simulink model "SAD_PROJECT"  (R2023b)
settings: Solver=ode5  StartTime=0.0  StopTime=5920  FixedStep=0.01  RelTol=1e-10  AbsTol=1e-11
values from neighbouring files (symbols this model uses):
  A = [0,  (1-K_yaw)*n, 0, -K_yaw*n^2,  0,   0 ... (first row only)    [SAD_CALLER.m]
  A_0 = A_B_LVLH*A_LVLH_ECI_0    [SAD_CALLER.m]    (also in veriAxilsym.m = eye(3))
  A_slew_B_LVLH = rot_matrix(deg2rad(-15.3),1)*rot_matrix(deg2rad(0),2)*rot_matrix(deg2rad(0),3)*eye(3)    [SAD_CALLER.m]
  alpha_mount_hs = 0.15    [SAD_CALLER.m]
  alpha_mount_ss = -0.5    [SAD_CALLER.m]
  B = [1/I(1,1),0,0 ... (first row only)    [SAD_CALLER.m]
  C = [0,0,0,1,0,0 ... (first row only)    [SAD_CALLER.m]
  correct_g = [5.7   7.4   0      0     0 ... (first row only)    [SAD_CALLER.m]    (also in veriAxilsym.m)
  correct_h = [  0  -25.9     0       0      0 ... (first row only)    [SAD_CALLER.m]    (also in veriAxilsym.m)
  d_cm_rw = 0.00000005    (= 5e-08)    [SAD_CALLER.m]
  d_cmsc_rw = 0.003    [SAD_CALLER.m]
  f = @(F) -F+e*sinh(F)+F_s-e*sinh(F_s)-M_h    [SAD_CALLER.m]
  FOV = 34    [SAD_CALLER.m]
  g_nm = [-29404.8 -1450.9     0      0     0 ... (first row only)    [SAD_CALLER.m]    (also in veriAxilsym.m)
  h_nm = [  0  4652.5      0      0       0 ... (first row only)    [SAD_CALLER.m]    (also in veriAxilsym.m)
  I = I_a+diag([0,4*M_a*x_cm^2,4*M_a*x_cm^2])+I_c+diag([0,M_c*d_cc_cm^2,M_c*d_cc_cm^2])+I_p+diag([0,6*M_p*(d_cc+d_cc_cm)^2,6*M_p*(d_cc-d_cc_cm)^2])    [SAD_CALLER.m]    (also in veriAxilsym.m = diag(I))
  I_r = 9.55e-5    (= 9.55e-05)    [SAD_CALLER.m]
  Inv_I = inv(I)    [SAD_CALLER.m]    (also in veriAxilsym.m = pinv(I))
  inv_R = inv(R)    [SAD_CALLER.m]
  J2 = 1.082626925638815e-3    (= 0.00108262692564)    [SAD_CALLER.m]    (also in veriAxilsym.m)
  K = [ -0.4323    0.0000   -0.0000   -0.0105    0.0000   -0.0000 ... (first row only)    [SAD_CALLER.m]
  L = [  0.0663    0.0001    0.0068 ... (first row only)    [SAD_CALLER.m]
  M_brake = 0.0002    [SAD_CALLER.m]
  M_rw = 0.2    [SAD_CALLER.m]    (also in veriAxilsym.m)
  m_sc_body = [1;1;1]*10e-3*M_tot/sqrt(3)    [SAD_CALLER.m]    (also in veriAxilsym.m)
  maneuver = input('type of maneuver, 1 for nadir pointing, 2 for de-tumbling, 3 for slew ')    [SAD_CALLER.m]
  mu_E = 3.986004418e5    (= 398600.4418)    [SAD_CALLER.m]    (also in veriAxilsym.m = 398600)
  mu_S = 1.327124400e11    (= 132712440000)    [SAD_CALLER.m]
  n = 2*pi/T    [SAD_CALLER.m]
  om_rw_0 = [0,0,0]    [SAD_CALLER.m]
  omega_E = 2*pi/(24*60*60)    (= 7.27220521664e-05)    [SAD_CALLER.m]    (also in veriAxilsym.m)
  omega_sc_0 = [0,0,n]    [SAD_CALLER.m]    (also in veriAxilsym.m = [0; 0; 0])
  pinv_R_xy = pinv(R_xy)    [SAD_CALLER.m]
  pinv_R_xz = pinv(R_xz)    [SAD_CALLER.m]
  pinv_R_yz = pinv(R_yz)    [SAD_CALLER.m]
  R = [cos(angle),-sin(angle),0;sin(angle),cos(angle),0;0,0,1]    [SAD_CALLER.m]    (also in veriAxilsym.m = 6378.1363)
  R_E_eqtr = 6378.1363    [SAD_CALLER.m]    (also in veriAxilsym.m)
  R_x = R(:,1)    [SAD_CALLER.m]
  R_y = R(:,2)    [SAD_CALLER.m]
  R_z = R(:,3)    [SAD_CALLER.m]
  rr_Esc_0 = s(end,(1:3))'    [SAD_CALLER.m]    (also in veriAxilsym.m = [7070.6; 0; 0])
  RR_x = [R_x,R_rad_x_1',R_rad_x_2']    [SAD_CALLER.m]
  RR_y = [R_y,R_rad_y_1',R_rad_y_2']    [SAD_CALLER.m]
  RR_z = [R_z,R_rad_z_1',R_rad_z_2']    [SAD_CALLER.m]
  smith_norm = zeros(4,5)    [SAD_CALLER.m]    (also in veriAxilsym.m)
  theta_G0 = mod(theta_G_Winter_solstice+omega_E*t_elapsed,2*pi)    [SAD_CALLER.m]    (also in veriAxilsym.m)
  vv_Esc_0 = s(end,(4:6))'    [SAD_CALLER.m]    (also in veriAxilsym.m = [0; 7.4338; 0])
undefined symbols (not defined in the file or in its folder): omega_0, rr_ES_0, vv_ES_0
libraries: matrix_library x24, simulink_extras x9, simulink x5
(part 1 of 2)
settings Model: Creator=WinUser  LastModifiedBy=a1pab

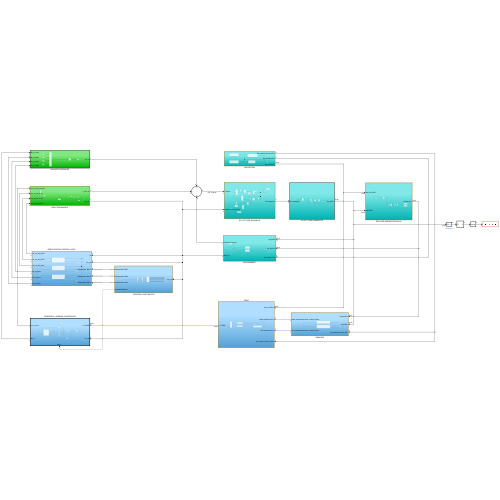
[thumbnail: Simulink's stored preview of the top-level diagram]
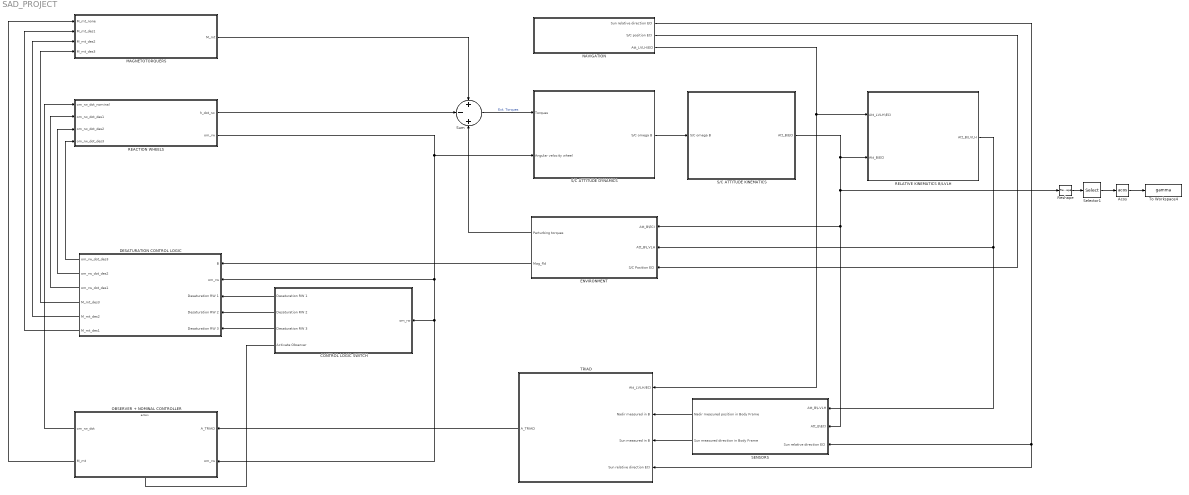
== system SAD_PROJECT ==
  Acos : Trigonometry  Operator=acos
  CONTROL LOGIC SWITCH : Subsystem
  DESATURATION CONTROL LOGIC : Subsystem
  ENVIRONMENT : Subsystem
  MAGNETOTORQUERS : Subsystem
  NAVIGATION : Subsystem
  OBSERVER + NOMINAL CONTROLLER : Subsystem  TreatAsAtomicUnit=on
  REACTION WHEELS : Subsystem
  RELATIVE KINEMATICS B/LVLH : Subsystem
  Reshape : Reshape
  S/C ATTITUDE DYNAMICS : Subsystem
  S/C ATTITUDE KINEMATICS : Subsystem
  SENSORS : Subsystem
  Selector1 : Selector  InputPortWidth=9  IndexOptions=Index vector (dialog)  Indices=[1,5,9]  OutputSizes=1
  Sum : Sum  Inputs=+-+
  TRIAD : Subsystem
  To Workspace4 : ToWorkspace  VariableName=gamma  SampleTime=-1
      settings: Save2DSignal=2-D array (concatenate along first dimension)
  wires:
  Sum/1 -> S/C ATTITUDE DYNAMICS/1(Torques)  "Ext. Torques"
  S/C ATTITUDE KINEMATICS/1(Att_B\ECI) -> Reshape/1, SENSORS/2(Att_B\ECI), ENVIRONMENT/1(Att_B\ECI), RELATIVE KINEMATICS B/LVLH/2(Att_B\ECI)
  ENVIRONMENT/1(Perturbing torques) -> Sum/3
  RELATIVE KINEMATICS B/LVLH/1(Att_B\LVLH) -> ENVIRONMENT/2(Att_B\LVLH), SENSORS/1(Att_B\LVLH)
  NAVIGATION/1(Sun relative direction ECI) -> TRIAD/4(Sun relative direction ECI), SENSORS/3(Sun relative direction ECI)
  NAVIGATION/3(Att_LVLH\ECI) -> TRIAD/1(Att_LVLH/ECI), RELATIVE KINEMATICS B/LVLH/1(Att_LVLH\ECI)
  NAVIGATION/2(S/C position ECI) -> ENVIRONMENT/3(S/C Position ECI)
  REACTION WHEELS/1(h_dot_rw) -> Sum/2
  ENVIRONMENT/2(Mag_fld) -> DESATURATION CONTROL LOGIC/1(B)
  SENSORS/1(Nadir measured position in Body Frame) -> TRIAD/2(Nadir measured in B)
  SENSORS/2(Sun measured direction in Body Frame) -> TRIAD/3(Sun measured in B)
  REACTION WHEELS/2(om_rw) -> OBSERVER + NOMINAL CONTROLLER/2(om_rw), CONTROL LOGIC SWITCH/1(om_rw), DESATURATION CONTROL LOGIC/2(om_rw), S/C ATTITUDE DYNAMICS/2(Angular velocity wheel)
  CONTROL LOGIC SWITCH/4(Activate Observer) -> OBSERVER + NOMINAL CONTROLLER/Action
  CONTROL LOGIC SWITCH/1(Desaturation RW 1) -> DESATURATION CONTROL LOGIC/3(Desaturation RW 1)
  CONTROL LOGIC SWITCH/2(Desaturation RW 2) -> DESATURATION CONTROL LOGIC/4(Desaturation RW 2)
  CONTROL LOGIC SWITCH/3(Desaturation RW 3) -> DESATURATION CONTROL LOGIC/5(Desaturation RW 3)
  OBSERVER + NOMINAL CONTROLLER/1(om_rw_dot) -> REACTION WHEELS/1(om_rw_dot_nominal)
  DESATURATION CONTROL LOGIC/3(om_rw_dot_des1) -> REACTION WHEELS/2(om_rw_dot_des1)
  DESATURATION CONTROL LOGIC/2(om_rw_dot_des2) -> REACTION WHEELS/3(om_rw_dot_des2)
  DESATURATION CONTROL LOGIC/1(om_rw_dot_des3) -> REACTION WHEELS/4(om_rw_dot_des3)
  DESATURATION CONTROL LOGIC/4(M_mt_des3) -> MAGNETOTORQUERS/4(M_mt_des3)
  DESATURATION CONTROL LOGIC/5(M_mt_des2) -> MAGNETOTORQUERS/3(M_mt_des2)
  DESATURATION CONTROL LOGIC/6(M_mt_des1) -> MAGNETOTORQUERS/2(M_mt_des1)
  MAGNETOTORQUERS/1(M_mt) -> Sum/1
  OBSERVER + NOMINAL CONTROLLER/2(M_mt) -> MAGNETOTORQUERS/1(M_mt_none)
  TRIAD/1(A_TRIAD) -> OBSERVER + NOMINAL CONTROLLER/1(A_TRIAD)
  S/C ATTITUDE DYNAMICS/1(S/C omega B) -> S/C ATTITUDE KINEMATICS/1(S/C omega B)
  Selector1/1 -> Acos/1
  Reshape/1 -> Selector1/1
  Acos/1 -> To Workspace4/1

== system SAD_PROJECT/CONTROL LOGIC SWITCH ==
  om_rw : Inport
  Abs : Abs  SaturateOnIntegerOverflow=off
  Abs1 : Abs  SaturateOnIntegerOverflow=off
  Abs2 : Abs  SaturateOnIntegerOverflow=off
  Demux : Demux  Outputs=3
  If : If  NumInputs=3  IfExpression=u1 == 1  ElseIfExpressions=u2== 1,u3==1
  Relay : Relay  OnSwitchValue=500  OffSwitchValue=100
  Relay1 : Relay  OnSwitchValue=500  OffSwitchValue=100
  Relay2 : Relay  OnSwitchValue=500  OffSwitchValue=100
  Desaturation RW 1 : Outport
  Desaturation RW 2 : Outport  Port=2
  Desaturation RW 3 : Outport  Port=3
  Activate Observer : Outport  Port=4
  wires:
  Demux/3 -> Abs2/1
  Demux/1 -> Abs/1
  Abs/1 -> Relay/1
  Demux/2 -> Abs1/1
  Abs2/1 -> Relay2/1
  Relay1/1 -> If/2
  Abs1/1 -> Relay1/1
  Relay/1 -> If/1
  Relay2/1 -> If/3
  If/1 -> Desaturation RW 1/1
  If/4 -> Activate Observer/1
  If/2 -> Desaturation RW 2/1
  om_rw/1 -> Demux/1
  If/3 -> Desaturation RW 3/1

== system SAD_PROJECT/DESATURATION CONTROL LOGIC ==
  B : Inport
  om_rw : Inport  Port=2
  Desaturation RW 1 : Inport  Port=3
  Desaturation RW 2 : Inport  Port=4
  Desaturation RW 3 : Inport  Port=5
  RW 1 Desaturation : Subsystem
  RW 2 Desaturation : Subsystem
  RW 3 Desaturation : Subsystem
  om_rw_dot_des3 : Outport
  om_rw_dot_des2 : Outport  Port=2
  om_rw_dot_des1 : Outport  Port=3
  M_mt_des3 : Outport  Port=4
  M_mt_des2 : Outport  Port=5
  M_mt_des1 : Outport  Port=6
  wires:
  Desaturation RW 1/1 -> RW 1 Desaturation/Action
  B/1 -> RW 3 Desaturation/1(B), RW 2 Desaturation/1(B), RW 1 Desaturation/1(B)
  Desaturation RW 2/1 -> RW 2 Desaturation/Action
  Desaturation RW 3/1 -> RW 3 Desaturation/Action
  om_rw/1 -> RW 3 Desaturation/2(om_rw), RW 2 Desaturation/2(om_rw), RW 1 Desaturation/2(om_rw)
  RW 1 Desaturation/1(M_mt) -> M_mt_des1/1
  RW 1 Desaturation/2(om_rw_dot) -> om_rw_dot_des1/1
  RW 2 Desaturation/1(M_mt) -> M_mt_des2/1
  RW 2 Desaturation/2(om_rw_dot) -> om_rw_dot_des2/1
  RW 3 Desaturation/1(M_mt) -> M_mt_des3/1
  RW 3 Desaturation/2(om_rw_dot) -> om_rw_dot_des3/1

== system SAD_PROJECT/ENVIRONMENT ==
  Att_B\ECI : Inport
  Att_B\LVLH : Inport  Port=2
  S/C Position ECI : Inport  Port=3
  Gravity Gradient : Subsystem
  Magnetic Torque : Subsystem
  Sum : Sum  Inputs=+|+
  To Workspace1 : ToWorkspace  VariableName=ext_perturbations  SampleTime=-1
  Perturbing torques : Outport
  Mag_fld : Outport  Port=2
  wires:
  S/C Position ECI/1 -> Gravity Gradient/2(S/C Position), Magnetic Torque/1("[km]")
  Att_B\ECI/1 -> Magnetic Torque/2(True Attitude B\N)
  Att_B\LVLH/1 -> Gravity Gradient/1(Att_B\L)
  Gravity Gradient/1(GG_Torque) -> Sum/1
  Sum/1 -> To Workspace1/1, Perturbing torques/1
  Magnetic Torque/1(MF_Torque) -> Sum/2
  Magnetic Torque/2(Mag_fld) -> Mag_fld/1

== system SAD_PROJECT/MAGNETOTORQUERS ==
  M_mt_none : Inport
  M_mt_des1 : Inport  Port=2
  M_mt_des2 : Inport  Port=3
  M_mt_des3 : Inport  Port=4
  Merge1 : Merge  Inputs=4
  Rate Limiter : RateLimiter  RisingSlewLimit=0.001  FallingSlewLimit=-0.001
  M_mt : Outport
  wires:
  Rate Limiter/1 -> M_mt/1
  Merge1/1 -> Rate Limiter/1
  M_mt_none/1 -> Merge1/1
  M_mt_des3/1 -> Merge1/4
  M_mt_des2/1 -> Merge1/3
  M_mt_des1/1 -> Merge1/2

== system SAD_PROJECT/NAVIGATION ==
  LVLH Kinematics : Subsystem
  S/C Orbit propagation : Subsystem
  Subsystem : Subsystem
  Sun orbit propagation : Subsystem
  Sun relative direction ECI : Outport
  S/C position ECI : Outport  Port=2
  Att_LVLH\ECI : Outport  Port=3
  wires:
  S/C Orbit propagation/1(S/C Posiion ECI) -> Subsystem/2(S/C position in ECI), S/C position ECI/1, LVLH Kinematics/1(position)
  Subsystem/1(Sun relative direction in ECI) -> Sun relative direction ECI/1
  Sun orbit propagation/1(Sun position in ECI) -> Subsystem/1(Sun position in ECI)
  S/C Orbit propagation/2(S/C Velocity ECI) -> LVLH Kinematics/2(velocity)  "[km/s]"
  LVLH Kinematics/1(Att_LVLH\ECI) -> Att_LVLH\ECI/1

== system SAD_PROJECT/OBSERVER + NOMINAL CONTROLLER ==
  A_TRIAD : Inport
  om_rw : Inport  Port=2
  Action Port : ActionPort  ActionPortLabel=else
  Gain : Gain  Gain=A  Multiplication=Matrix(K*u) (u vector)
  Gain1 : Gain  Gain=B  Multiplication=Matrix(K*u) (u vector)
  Gain2 : Gain  Gain=C  Multiplication=Matrix(K*u) (u vector)
  Gain3 : Gain  Gain=L  Multiplication=Matrix(K*u) (u vector)
  Integrator : Integrator
  NOMINAL CONTROL : Subsystem
  Reshape1 : Reshape
  Selector1 : Selector  InputPortWidth=9  IndexOptions=Index vector (dialog)  Indices=[8,3,4]  OutputSizes=1
  Sum2 : Sum  Inputs=|+-
  Sum4 : Sum  Inputs=+++
  om_rw_dot : Outport
  M_mt : Outport  Port=2
  wires:
  Sum4/1 -> Integrator/1
  NOMINAL CONTROL/1(u) -> Gain1/1
  Gain1/1 -> Sum4/1
  Gain3/1 -> Sum4/2
  Gain/1 -> Sum4/3
  Sum2/1 -> Gain3/1
  Gain2/1 -> Sum2/2
  Integrator/1 -> Gain/1, Gain2/1, NOMINAL CONTROL/1(x_hat)  "x_hat"
  om_rw/1 -> NOMINAL CONTROL/2(om_rw)
  NOMINAL CONTROL/2(om_rw_dot) -> om_rw_dot/1
  NOMINAL CONTROL/3(M_mt) -> M_mt/1
  A_TRIAD/1 -> Reshape1/1
  Reshape1/1 -> Selector1/1
  Selector1/1 -> Sum2/1  "[alpha_x,alpha_y,alpha_z"

== system SAD_PROJECT/REACTION WHEELS ==
  om_rw_dot_nominal : Inport
  om_rw_dot_des1 : Inport  Port=2
  om_rw_dot_des2 : Inport  Port=3
  om_rw_dot_des3 : Inport  Port=4
  Band-Limited White Noise : simulink/Sources/Band-Limited White Noise  Cov=[0.1]  Ts=0.1  seed=[23341]
  Constant1 : Constant  Value=om_rw_0
  Constant5 : Constant  Value=[I_r;I_r;I_r]
  Constant7 : Constant  Value=R
  Gain : Gain  Gain=1.74
  Integrator : Integrator  InitialConditionSource=external
  Matrix Multiply4 : Product
  Matrix Multiply7 : Product  Multiplication=Matrix(*)
  Merge : Merge  Inputs=4
  Rate Limiter1 : RateLimiter  RisingSlewLimit=0.001  FallingSlewLimit=-0.001  SampleTimeMode=inherited
  Saturation : Saturate  UpperLimit=125  LowerLimit=-125
  Subsystem1 : Subsystem
  Sum : Sum  Inputs=++|
  Sum1 : Sum  Inputs=|+-
  To Workspace : ToWorkspace  VariableName=rw_perturbations  SaveFormat=Timeseries  SampleTime=-1
  Transfer Fcn : TransferFcn  Denominator=[10 1]
  h_dot_rw : Outport
  om_rw : Outport  Port=2
  wires:
  Constant5/1 -> Matrix Multiply4/1
  Constant7/1 -> Matrix Multiply7/1
  Sum/1 -> Subsystem1/1(om_rw), om_rw/1  "om_rw"
  Merge/1 -> Saturation/1  "om_dot_rw"
  Matrix Multiply4/1 -> Matrix Multiply7/2  "h_dot_rw"
  Constant1/1 -> Integrator/2
  Matrix Multiply7/1 -> Rate Limiter1/1
  om_rw_dot_nominal/1 -> Merge/1  "om_dot_rw"
  Rate Limiter1/1 -> Sum1/1
  Saturation/1 -> Matrix Multiply4/2, Integrator/1
  Band-Limited White Noise/1 -> Gain/1
  Gain/1 -> Transfer Fcn/1
  Integrator/1 -> Sum/2  "om_rw"
  Subsystem1/1(disturbance torque) -> To Workspace/1, Sum1/2
  Sum1/1 -> h_dot_rw/1
  Transfer Fcn/1 -> Sum/1
  om_rw_dot_des1/1 -> Merge/2
  om_rw_dot_des2/1 -> Merge/3
  om_rw_dot_des3/1 -> Merge/4

== system SAD_PROJECT/RELATIVE KINEMATICS B//LVLH ==
  Att_LVLH\ECI : Inport
  Att_B\ECI : Inport  Port=2
  Acos : Trigonometry  Operator=acos
  Demux : Demux  Outputs=2
  Matrix Multiply1 : Product  Multiplication=Matrix(*)
  Radians to Degrees : simulink_extras/Transformations/Radians to Degrees
  Reshape : Reshape
  Selector : Selector  InputPortWidth=9  IndexOptions=Index vector (dialog)  Indices=[1,9]  OutputSizes=1
  To Workspace2 : ToWorkspace  VariableName=alpha_x  SampleTime=-1
      settings: Save2DSignal=2-D array (concatenate along first dimension)
  To Workspace3 : ToWorkspace  VariableName=alpha_z  SampleTime=-1
      settings: Save2DSignal=2-D array (concatenate along first dimension)
  Transpose1 : Math  Operator=transpose
  Att_B\LVLH : Outport
  wires:
  Transpose1/1 -> Matrix Multiply1/2  "A_N\\L"
  Matrix Multiply1/1 -> Reshape/1, Att_B\LVLH/1  "A B\\L"
  Att_B\ECI/1 -> Matrix Multiply1/1
  Att_LVLH\ECI/1 -> Transpose1/1
  Demux/2 -> To Workspace3/1
  Demux/1 -> To Workspace2/1
  Selector/1 -> Acos/1
  Reshape/1 -> Selector/1
  Radians to Degrees/1 -> Demux/1
  Acos/1 -> Radians to Degrees/1

== system SAD_PROJECT/S//C ATTITUDE DYNAMICS ==
  note: omega
  Torques : Inport
  Angular velocity wheel : Inport  Port=2
  Constant : Constant  Value=omega_sc_0
  Constant1 : Constant  Value=I  VectorParams1D=off
  Constant2 : Constant  Value=R
  Constant3 : Constant  Value=Inv_I  VectorParams1D=off
  Constant4 : Constant  Value=[I_r;I_r;I_r]
  Cross Product : matrix_library/Cross Product
  Integrator : Integrator  InitialConditionSource=external  InitialCondition=omega_0
  Matrix Multiply : Product  Multiplication=Matrix(*)
  Matrix Multiply1 : Product
  Matrix Multiply2 : Product  Multiplication=Matrix(*)
  Product : Product  Multiplication=Matrix(*)
  Sum : Sum  Inputs=|+-
  Sum1 : Sum  Inputs=|++
  To Workspace : ToWorkspace  VariableName=omega_rw  SampleTime=-1
  To Workspace4 : ToWorkspace  VariableName=omega_sc  SampleTime=-1
  S/C omega B : Outport
  wires:
  Constant3/1 -> Matrix Multiply/1
  Constant/1 -> Integrator/2
  Sum/1 -> Matrix Multiply/2
  Cross Product/1 -> Sum/2
  Integrator/1 -> To Workspace4/1, S/C omega B/1, Cross Product/1, Product/2
  Constant1/1 -> Product/1
  Matrix Multiply/1 -> Integrator/1
  Torques/1 -> Sum/1
  Angular velocity wheel/1 -> To Workspace/1, Matrix Multiply1/2
  Constant2/1 -> Matrix Multiply2/1
  Product/1 -> Sum1/1
  Sum1/1 -> Cross Product/2
  Matrix Multiply2/1 -> Sum1/2
  Constant4/1 -> Matrix Multiply1/1
  Matrix Multiply1/1 -> Matrix Multiply2/2

== system SAD_PROJECT/S//C ATTITUDE KINEMATICS ==
  S/C omega B : Inport
  1st order orthon. : Subsystem
  Angular velocity tensor : Subsystem
  Constant3 : Constant  Value=A_0
  Gain : Gain  Gain=-1
  Integrator1 : Integrator  InitialConditionSource=external  InitialCondition=omega_0
  Matrix Multiply : Product  Multiplication=Matrix(*)
  Att_B\ECI : Outport
  wires:
  Constant3/1 -> Integrator1/2
  S/C omega B/1 -> Angular velocity tensor/1(In1)  "omega B\\N"
  1st order orthon./1(Out1) -> Att_B\ECI/1, Matrix Multiply/2  "True Attitude B\\N"
  Integrator1/1 -> 1st order orthon./1(In1)
  Matrix Multiply/1 -> Integrator1/1
  Gain/1 -> Matrix Multiply/1
  Angular velocity tensor/1(Out1) -> Gain/1

== system SAD_PROJECT/SENSORS ==
  Att_B\LVLH : Inport
  Att_B\ECI : Inport  Port=2
  Sun relative direction ECI : Inport  Port=3
  Horizon Sensor : Subsystem
  Sun Sensor : Subsystem
  Nadir measured position in Body Frame : Outport
  Sun measured direction in Body Frame : Outport  Port=2
  wires:
  Att_B\ECI/1 -> Sun Sensor/1(Attitude B\ECI)
  Att_B\LVLH/1 -> Horizon Sensor/1(Attitude B\L)
  Sun relative direction ECI/1 -> Sun Sensor/2(Sun relative direction in ECI)
  Horizon Sensor/1(Nadir measured position in Body Frame) -> Nadir measured position in Body Frame/1
  Sun Sensor/1(Sun measured direction in Body Frame) -> Sun measured direction in Body Frame/1

== system SAD_PROJECT/TRIAD ==
  Att_LVLH/ECI : Inport
  Nadir measured in B : Inport  Port=2
  Sun measured in B : Inport  Port=3
  Sun relative direction ECI : Inport  Port=4
  Constant : Constant  Value=[1;0;0]
  Matrix Multiply : Product  Multiplication=Matrix(*)
  Subsystem : Subsystem
  Subsystem1 : Subsystem
  Subsystem2 : Subsystem
  Zero-Order Hold : ZeroOrderHold  SampleTime=0.2
  A_TRIAD : Outport
  wires:
  Sun relative direction ECI/1 -> Subsystem1/2(Sun relative direction ECI)
  Matrix Multiply/1 -> A_TRIAD/1
  Att_LVLH/ECI/1 -> Subsystem1/1(Att_LVLH/ECI)
  Nadir measured in B/1 -> Subsystem/1(a)
  Sun measured in B/1 -> Subsystem/2(b)
  Subsystem/1(Measures in Body) -> Matrix Multiply/1
  Constant/1 -> Subsystem2/1(Nadir in LVLH)  "Nadir in LVLH"
  Subsystem1/1(Sun direction in LVLH) -> Subsystem2/2(Sun in LVLH)  "Sun in LVLH"
  Subsystem2/1(Out1) -> Zero-Order Hold/1
  Zero-Order Hold/1 -> Matrix Multiply/2

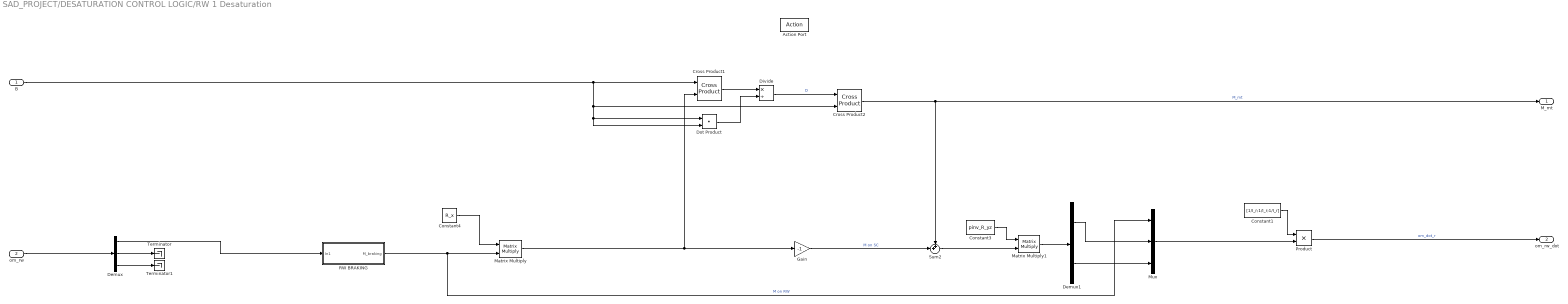
== system SAD_PROJECT/DESATURATION CONTROL LOGIC/RW 1 Desaturation ==
  B : Inport
  om_rw : Inport  Port=2
  Action Port : ActionPort  ActionPortLabel=if(u1 == 1)
  Constant1 : Constant  Value=[1/I_r;1/I_r;1/I_r]
  Constant3 : Constant  Value=pinv_R_yz
  Constant4 : Constant  Value=R_x
  Cross Product1 : matrix_library/Cross Product
  Cross Product2 : matrix_library/Cross Product
  Demux : Demux  Outputs=3
  Demux1 : Demux  Outputs=2
  Divide : Product  Inputs=*/
  Dot Product : DotProduct  OutDataTypeStr=Inherit: Inherit via internal rule
  Gain : Gain  Gain=-1
  Matrix Multiply : Product  Multiplication=Matrix(*)
  Matrix Multiply1 : Product  Multiplication=Matrix(*)
  Mux : Mux  Inputs=3
  Product : Product
  RW BRAKING : Subsystem
  Sum2 : Sum  Inputs=++|
  Terminator : Terminator
  Terminator1 : Terminator
  M_mt : Outport
  om_rw_dot : Outport  Port=2
  wires:
  Product/1 -> om_rw_dot/1  "om_dot_r"
  Cross Product2/1 -> Sum2/1, M_mt/1  "M_mt"
  Demux/3 -> Terminator1/1
  Constant3/1 -> Matrix Multiply1/1
  Matrix Multiply1/1 -> Demux1/1
  Constant4/1 -> Matrix Multiply/1
  Mux/1 -> Product/2
  Dot Product/1 -> Divide/2
  Demux1/2 -> Mux/3
  Demux/1 -> RW BRAKING/1(In1)
  Sum2/1 -> Matrix Multiply1/2
  Constant1/1 -> Product/1
  Divide/1 -> Cross Product2/1  "D"
  B/1 -> Dot Product/1, Dot Product/2, Cross Product2/2, Cross Product1/1
  RW BRAKING/1(M_braking) -> Mux/1, Matrix Multiply/2  "M on RW"
  om_rw/1 -> Demux/1
  Matrix Multiply/1 -> Gain/1, Cross Product1/2
  Cross Product1/1 -> Divide/1
  Gain/1 -> Sum2/2  "M on SC"
  Demux/2 -> Terminator/1
  Demux1/1 -> Mux/2

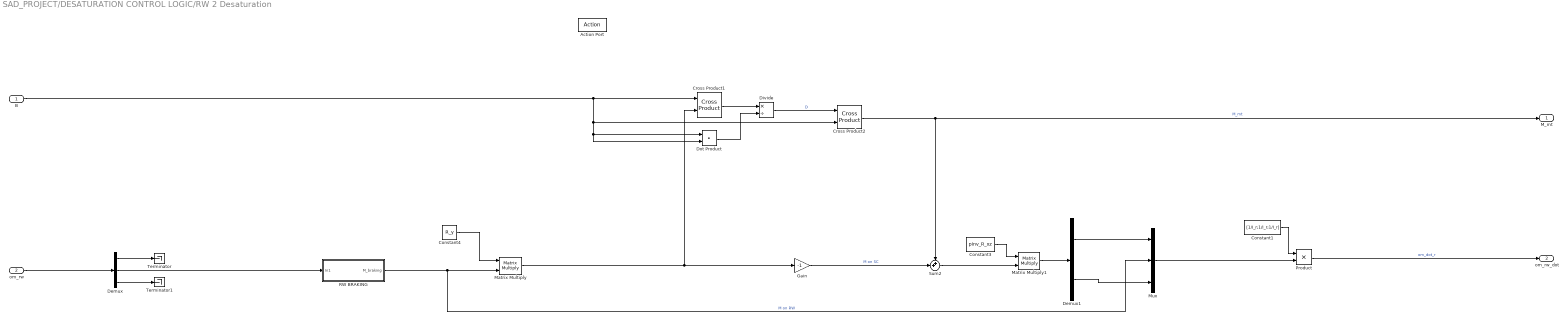
== system SAD_PROJECT/DESATURATION CONTROL LOGIC/RW 2 Desaturation ==
  B : Inport
  om_rw : Inport  Port=2
  Action Port : ActionPort  ActionPortLabel=elseif(u2== 1)
  Constant1 : Constant  Value=[1/I_r;1/I_r;1/I_r]
  Constant3 : Constant  Value=pinv_R_xz
  Constant4 : Constant  Value=R_y
  Cross Product1 : matrix_library/Cross Product
  Cross Product2 : matrix_library/Cross Product
  Demux : Demux  Outputs=3
  Demux1 : Demux  Outputs=2
  Divide : Product  Inputs=*/
  Dot Product : DotProduct  OutDataTypeStr=Inherit: Inherit via internal rule
  Gain : Gain  Gain=-1
  Matrix Multiply : Product  Multiplication=Matrix(*)
  Matrix Multiply1 : Product  Multiplication=Matrix(*)
  Mux : Mux  Inputs=3
  Product : Product
  RW BRAKING : Subsystem
  Sum2 : Sum  Inputs=++|
  Terminator : Terminator
  Terminator1 : Terminator
  M_mt : Outport
  om_rw_dot : Outport  Port=2
  wires:
  Demux1/1 -> Mux/1
  Cross Product2/1 -> Sum2/1, M_mt/1  "M_mt"
  B/1 -> Dot Product/1, Dot Product/2, Cross Product2/2, Cross Product1/1
  Dot Product/1 -> Divide/2
  Constant4/1 -> Matrix Multiply/1
  Divide/1 -> Cross Product2/1  "D"
  Cross Product1/1 -> Divide/1
  RW BRAKING/1(M_braking) -> Mux/2, Matrix Multiply/2  "M on RW"
  Demux1/2 -> Mux/3
  Gain/1 -> Sum2/2  "M on SC"
  Sum2/1 -> Matrix Multiply1/2
  Constant3/1 -> Matrix Multiply1/1
  om_rw/1 -> Demux/1
  Demux/2 -> RW BRAKING/1(In1)
  Demux/3 -> Terminator1/1
  Demux/1 -> Terminator/1
  Constant1/1 -> Product/1
  Product/1 -> om_rw_dot/1  "om_dot_r"
  Mux/1 -> Product/2
  Matrix Multiply1/1 -> Demux1/1
  Matrix Multiply/1 -> Gain/1, Cross Product1/2

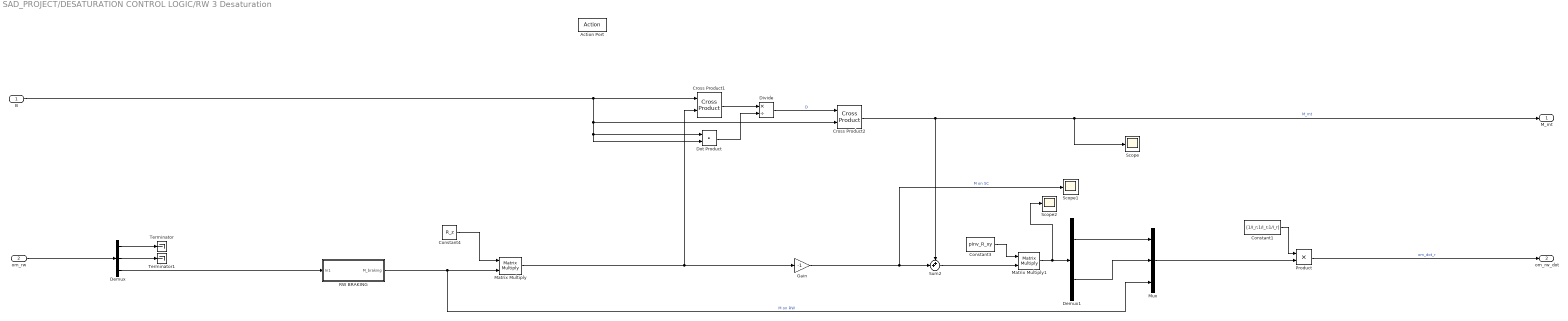
== system SAD_PROJECT/DESATURATION CONTROL LOGIC/RW 3 Desaturation ==
  B : Inport
  om_rw : Inport  Port=2
  Action Port : ActionPort  ActionPortLabel=elseif(u3==1)
  Constant1 : Constant  Value=[1/I_r;1/I_r;1/I_r]
  Constant3 : Constant  Value=pinv_R_xy
  Constant4 : Constant  Value=R_z
  Cross Product1 : matrix_library/Cross Product
  Cross Product2 : matrix_library/Cross Product
  Demux : Demux  Outputs=3
  Demux1 : Demux  Outputs=2
  Divide : Product  Inputs=*/
  Dot Product : DotProduct  OutDataTypeStr=Inherit: Inherit via internal rule
  Gain : Gain  Gain=-1
  Matrix Multiply : Product  Multiplication=Matrix(*)
  Matrix Multiply1 : Product  Multiplication=Matrix(*)
  Mux : Mux  Inputs=3
  Product : Product
  RW BRAKING : Subsystem
  Scope : Scope
  Scope1 : Scope
  Scope2 : Scope
  Sum2 : Sum  Inputs=++|
  Terminator : Terminator
  Terminator1 : Terminator
  M_mt : Outport
  om_rw_dot : Outport  Port=2
  wires:
  Demux1/1 -> Mux/1
  Cross Product2/1 -> Sum2/1, Scope/1, M_mt/1  "M_mt"
  B/1 -> Dot Product/1, Dot Product/2, Cross Product2/2, Cross Product1/1
  Dot Product/1 -> Divide/2
  Constant4/1 -> Matrix Multiply/1
  Divide/1 -> Cross Product2/1  "D"
  Cross Product1/1 -> Divide/1
  RW BRAKING/1(M_braking) -> Mux/3, Matrix Multiply/2  "M on RW"
  Demux1/2 -> Mux/2
  Gain/1 -> Scope1/1, Sum2/2  "M on SC"
  Sum2/1 -> Matrix Multiply1/2
  Constant3/1 -> Matrix Multiply1/1
  om_rw/1 -> Demux/1
  Demux/3 -> RW BRAKING/1(In1)
  Demux/1 -> Terminator/1
  Constant1/1 -> Product/1
  Product/1 -> om_rw_dot/1  "om_dot_r"
  Mux/1 -> Product/2
  Matrix Multiply1/1 -> Scope2/1, Demux1/1
  Matrix Multiply/1 -> Gain/1, Cross Product1/2
  Demux/2 -> Terminator1/1

== system SAD_PROJECT/ENVIRONMENT/Gravity Gradient ==
  Att_B\L : Inport
  S/C Position : Inport  Port=2
  Constant : Constant  Value=-1.5
  Constant7 : Constant  Value=I
  Constant8 : Constant  Value=0
  Demux : Demux  Outputs=2
  Dot Product : DotProduct  OutDataTypeStr=Inherit: Inherit via internal rule
  Gain2 : Gain  Gain=3*mu_E
  Gain3 : Gain  Gain=-1
  Matrix Multiply5 : Product  Multiplication=Matrix(*)
  Mux4 : Mux  Inputs=3
  Power : Math  Operator=pow
  Product : Product
  Reshape : Reshape
  Selector : Selector  InputPortWidth=9  IndexOptions=Index vector (dialog)  Indices=[2,3]  OutputSizes=1
  Subsystem : Subsystem
  GG_Torque : Outport
  wires:
  Selector/1 -> Demux/1
  Reshape/1 -> Selector/1
  Att_B\L/1 -> Subsystem/1(Att_B\L), Matrix Multiply5/1
  Mux4/1 -> Gain2/1
  Constant8/1 -> Mux4/1
  Demux/1 -> Mux4/3
  Matrix Multiply5/1 -> GG_Torque/1
  Demux/2 -> Gain3/1
  Gain3/1 -> Mux4/2
  Constant7/1 -> Subsystem/2(I_Body)
  Subsystem/1(I LVLH FRAME) -> Reshape/1
  Gain2/1 -> Product/1
  Product/1 -> Matrix Multiply5/2
  S/C Position/1 -> Dot Product/1, Dot Product/2
  Dot Product/1 -> Power/1
  Constant/1 -> Power/2
  Power/1 -> Product/2

== system SAD_PROJECT/ENVIRONMENT/Magnetic Torque ==
  "[km]" : Inport
  True Attitude B\N : Inport  Port=2
  Cartesian 2 spherical : Subsystem
  Constant1 : Constant  Value=m_sc_body
  MAGNETIC TORQUE in BODY : Subsystem
  MF_Torque : Outport
  Mag_fld : Outport  Port=2
  wires:
  "[km]"/1 -> Cartesian 2 spherical/1("[km]")
  Cartesian 2 spherical/1(LST) -> MAGNETIC TORQUE in BODY/1(local siderial time)
  Cartesian 2 spherical/2(Long) -> MAGNETIC TORQUE in BODY/2(longitude)  "[rad]"
  Cartesian 2 spherical/3(radius) -> MAGNETIC TORQUE in BODY/3(r)
  Constant1/1 -> MAGNETIC TORQUE in BODY/6(a)
  MAGNETIC TORQUE in BODY/1(M) -> MF_Torque/1
  Cartesian 2 spherical/4(lat) -> MAGNETIC TORQUE in BODY/4(latitude)  "[rad]"
  True Attitude B\N/1 -> MAGNETIC TORQUE in BODY/5(True_Att_B\N)
  MAGNETIC TORQUE in BODY/2(Mag_fld) -> Mag_fld/1

== system SAD_PROJECT/NAVIGATION/LVLH Kinematics ==
  position : Inport
  velocity : Inport  Port=2
  Cross Product : matrix_library/Cross Product
  Cross Product1 : matrix_library/Cross Product
  Divide : Product  Inputs=*/
  Divide1 : Product  Inputs=*/
  Divide2 : Product  Inputs=*/
  Dot Product : DotProduct  OutDataTypeStr=Inherit: Inherit via internal rule
  Dot Product1 : DotProduct  OutDataTypeStr=Inherit: Inherit via internal rule
  Dot Product2 : DotProduct  OutDataTypeStr=Inherit: Inherit via internal rule
  Matrix Concatenate : Concatenate  NumInputs=3  Mode=Multidimensional array  ConcatenateDimension=2
  Sqrt : Sqrt
  Sqrt1 : Sqrt
  Sqrt2 : Sqrt
  Transpose : Math  Operator=transpose
  Att_LVLH\ECI : Outport
  wires:
  Divide2/1 -> Matrix Concatenate/2  "along track unit vector y"
  Sqrt/1 -> Divide/2
  Cross Product/1 -> Dot Product1/2, Dot Product1/1, Divide1/1, Cross Product1/1
  Cross Product1/1 -> Divide2/1, Dot Product2/1, Dot Product2/2  "along track"
  Divide/1 -> Matrix Concatenate/1  "position unit vector x"
  position/1 -> Divide/1, Dot Product/1, Dot Product/2, Cross Product1/2, Cross Product/1
  velocity/1 -> Cross Product/2
  Sqrt2/1 -> Divide1/2
  Matrix Concatenate/1 -> Transpose/1
  Sqrt1/1 -> Divide2/2
  Divide1/1 -> Matrix Concatenate/3  "angular momentum unit vector z"
  Dot Product1/1 -> Sqrt2/1
  Dot Product/1 -> Sqrt/1
  Dot Product2/1 -> Sqrt1/1
  Transpose/1 -> Att_LVLH\ECI/1  "Attitude L\\N"

== system SAD_PROJECT/NAVIGATION/S//C Orbit propagation ==
  Constant5 : Constant  Value=vv_Esc_0
  Constant6 : Constant  Value=rr_Esc_0
  Integrator2 : Integrator  InitialConditionSource=external
  Integrator3 : Integrator  InitialConditionSource=external
  J2 perturbation : Subsystem
  Keplerian motion : Subsystem
  Sum : Sum  Inputs=|+-
  To Workspace : ToWorkspace  VariableName=RR_Esc  SampleTime=-1
  To Workspace1 : ToWorkspace  VariableName=VV_Esc  SampleTime=-1
  S/C Posiion ECI : Outport
  S/C Velocity ECI : Outport  Port=2
  wires:
  J2 perturbation/1(J2 acceleration) -> Sum/1
  Keplerian motion/1(Keplerian acceleration) -> Sum/2
  Constant5/1 -> Integrator2/2
  Integrator2/1 -> To Workspace1/1, S/C Velocity ECI/1, Integrator3/1  "dr"
  Constant6/1 -> Integrator3/2
  Sum/1 -> Integrator2/1  "ddr"
  Integrator3/1 -> S/C Posiion ECI/1, J2 perturbation/1(Position vector), Keplerian motion/1(Position vector), To Workspace/1  "r"

== system SAD_PROJECT/NAVIGATION/Subsystem ==
  Sun position in ECI : Inport
  S/C position in ECI : Inport  Port=2
  Divide2 : Product  Inputs=*/
  Dot Product2 : DotProduct  OutDataTypeStr=Inherit: Inherit via internal rule
  Sqrt2 : Sqrt
  Sum1 : Sum  Inputs=|+-
  Sun relative direction in ECI : Outport
  wires:
  Sum1/1 -> Dot Product2/2, Dot Product2/1, Divide2/1
  Dot Product2/1 -> Sqrt2/1
  Sqrt2/1 -> Divide2/2
  S/C position in ECI/1 -> Sum1/2
  Sun position in ECI/1 -> Sum1/1
  Divide2/1 -> Sun relative direction in ECI/1

== system SAD_PROJECT/NAVIGATION/Sun orbit propagation ==
  Constant5 : Constant  Value=vv_ES_0
  Constant6 : Constant  Value=rr_ES_0
  Integrator2 : Integrator  InitialConditionSource=external
  Integrator3 : Integrator  InitialConditionSource=external
  Keplerian motion : Subsystem
  Sum2 : Sum  Inputs=|+-
  To Workspace : ToWorkspace  VariableName=RR_ES  SampleTime=-1
  To Workspace1 : ToWorkspace  VariableName=VV_ES  SampleTime=-1
  Sun position in ECI : Outport
  wires:
  Integrator2/1 -> To Workspace1/1, Integrator3/1  "dr"
  Sum2/1 -> Integrator2/1  "ddr"
  Constant6/1 -> Integrator3/2
  Constant5/1 -> Integrator2/2
  Keplerian motion/1(Keplerian acceleration) -> Sum2/2
  Integrator3/1 -> To Workspace/1, Sun position in ECI/1, Keplerian motion/1(Position vector)  "Sun relative direction in ECI"

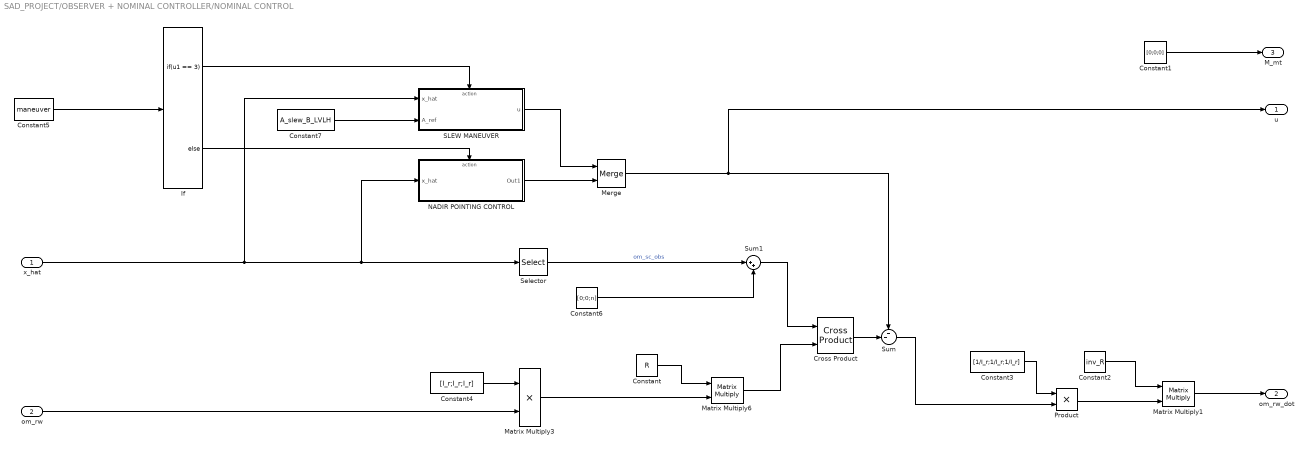
== system SAD_PROJECT/OBSERVER + NOMINAL CONTROLLER/NOMINAL CONTROL ==
  x_hat : Inport
  om_rw : Inport  Port=2
  Constant : Constant  Value=R
  Constant1 : Constant  Value=[0;0;0]
  Constant2 : Constant  Value=inv_R
  Constant3 : Constant  Value=[1/I_r;1/I_r;1/I_r]
  Constant4 : Constant  Value=[I_r;I_r;I_r]
  Constant5 : Constant  Value=maneuver
  Constant6 : Constant  Value=[0;0;n]
  Constant7 : Constant  Value=A_slew_B_LVLH
  Cross Product : matrix_library/Cross Product
  If : If  IfExpression=u1 == 3
  Matrix Multiply1 : Product  Multiplication=Matrix(*)
  Matrix Multiply3 : Product
  Matrix Multiply6 : Product  Multiplication=Matrix(*)
  Merge : Merge
  NADIR POINTING CONTROL : Subsystem  TreatAsAtomicUnit=on
  Product : Product
  SLEW MANEUVER : Subsystem  TreatAsAtomicUnit=on
  Selector : Selector  InputPortWidth=6  IndexOptions=Index vector (dialog)  Indices=[1 2 3]  OutputSizes=1
  Sum : Sum  Inputs=--|
  Sum1 : Sum  Inputs=|++
  u : Outport
  om_rw_dot : Outport  Port=2
  M_mt : Outport  Port=3
  wires:
  x_hat/1 -> SLEW MANEUVER/1(x_hat), NADIR POINTING CONTROL/1(x_hat), Selector/1
  Selector/1 -> Sum1/1  "om_sc_obs"
  Sum/1 -> Product/2
  Constant3/1 -> Product/1
  Matrix Multiply6/1 -> Cross Product/2
  Constant1/1 -> M_mt/1
  om_rw/1 -> Matrix Multiply3/2
  Constant6/1 -> Sum1/2
  Product/1 -> Matrix Multiply1/2
  Constant4/1 -> Matrix Multiply3/1
  Sum1/1 -> Cross Product/1
  Matrix Multiply1/1 -> om_rw_dot/1
  Constant2/1 -> Matrix Multiply1/1
  Cross Product/1 -> Sum/2
  Matrix Multiply3/1 -> Matrix Multiply6/2
  Constant/1 -> Matrix Multiply6/1
  Constant5/1 -> If/1
  Merge/1 -> u/1, Sum/1
  If/2 -> NADIR POINTING CONTROL/Action
  If/1 -> SLEW MANEUVER/Action
  Constant7/1 -> SLEW MANEUVER/2(A_ref)
  NADIR POINTING CONTROL/1(Out1) -> Merge/2
  SLEW MANEUVER/1(u) -> Merge/1

== system SAD_PROJECT/REACTION WHEELS/Subsystem1 ==
  om_rw : Inport
  Demux : Demux  Outputs=3
  Sum : Sum  Inputs=+++
  static unbalance rw1 : Subsystem
  static unbalance rw2 : Subsystem
  static unbalance rw3 : Subsystem
  disturbance torque : Outport
  wires:
  static unbalance rw1/1(Output) -> Sum/1
  Sum/1 -> disturbance torque/1
  static unbalance rw3/1(Output) -> Sum/3
  static unbalance rw2/1(Output) -> Sum/2
  Demux/1 -> static unbalance rw1/1(om_rw_1)  "om_rw_1"
  om_rw/1 -> Demux/1
  Demux/2 -> static unbalance rw2/1(om_rw_2)  "om_rw_2"
  Demux/3 -> static unbalance rw3/1(om_rw_1)  "om_rw_3"

== system SAD_PROJECT/S//C ATTITUDE KINEMATICS/1st order orthon. ==
  In1 : Inport
  Gain1 : Gain  Gain=3/2
  Gain2 : Gain  Gain=1/2
  Matrix Multiply1 : Product  Multiplication=Matrix(*)
  Matrix Multiply2 : Product  Multiplication=Matrix(*)
  Sum1 : Sum  Inputs=|+-
  Transpose : Math  Operator=transpose
  Out1 : Outport
  wires:
  Gain1/1 -> Sum1/1
  In1/1 -> Matrix Multiply2/2, Transpose/1, Gain2/1, Gain1/1
  Transpose/1 -> Matrix Multiply1/2
  Matrix Multiply2/1 -> Sum1/2
  Matrix Multiply1/1 -> Matrix Multiply2/1
  Sum1/1 -> Out1/1
  Gain2/1 -> Matrix Multiply1/1

== system SAD_PROJECT/S//C ATTITUDE KINEMATICS/Angular velocity tensor ==
  In1 : Inport
  Constant : Constant  Value=0
  Demux1 : Demux  Outputs=3
  Gain3 : Gain  Gain=-1
  Gain4 : Gain  Gain=-1
  Gain5 : Gain  Gain=-1
  Mux3 : Mux  Inputs=3
  Mux4 : Mux  Inputs=3
  Mux5 : Mux  Inputs=3
  Vector Concatenate : Concatenate  NumInputs=3  Mode=Multidimensional array  ConcatenateDimension=2
  Out1 : Outport
  wires:
  In1/1 -> Demux1/1
  Constant/1 -> Mux3/1, Mux4/2, Mux5/3
  Demux1/3 -> Gain4/1, Mux3/2
  Demux1/2 -> Gain3/1, Mux5/1
  Gain3/1 -> Mux3/3
  Gain4/1 -> Mux4/1
  Mux4/1 -> Vector Concatenate/2
  Demux1/1 -> Gain5/1, Mux4/3
  Gain5/1 -> Mux5/2
  Mux5/1 -> Vector Concatenate/3
  Mux3/1 -> Vector Concatenate/1
  Vector Concatenate/1 -> Out1/1

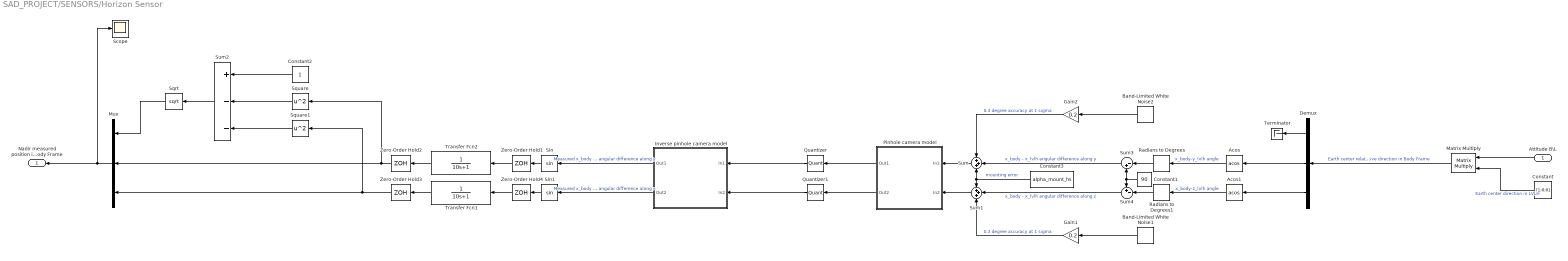
== system SAD_PROJECT/SENSORS/Horizon Sensor ==
  Attitude B\L : Inport
  Acos : Trigonometry  Operator=acos
  Acos1 : Trigonometry  Operator=acos
  Band-Limited White Noise1 : simulink/Sources/Band-Limited White Noise  Cov=[0.1]  Ts=0.1  seed=[23344]
  Band-Limited White Noise2 : simulink/Sources/Band-Limited White Noise  Cov=[0.1]  Ts=0.1  seed=[23344]
  Constant : Constant  Value=[1;0;0]
  Constant1 : Constant  Value=90
  Constant2 : Constant
  Constant3 : Constant  Value=alpha_mount_hs
  Demux : Demux  Outputs=3
  Gain1 : Gain  Gain=0.2
  Gain2 : Gain  Gain=0.2
  Inverse pinhole camera model : Subsystem
  Matrix Multiply : Product  Multiplication=Matrix(*)
  Mux : Mux  Inputs=3
  Pinhole camera model : Subsystem
  Quantizer : Quantizer  QuantizationInterval=0.2
  Quantizer1 : Quantizer  QuantizationInterval=0.2
  Radians to Degrees : simulink_extras/Transformations/Radians to Degrees
  Radians to Degrees1 : simulink_extras/Transformations/Radians to Degrees
  Scope : Scope
  Sin : Trigonometry
  Sin1 : Trigonometry
  Sqrt : Sqrt
  Square : Math  Operator=square
  Square1 : Math  Operator=square
  Sum : Sum  Inputs=+++
  Sum1 : Sum  Inputs=+++
  Sum2 : Sum  Inputs=+--
  Sum3 : Sum  Inputs=|-+
  Sum4 : Sum  Inputs=+-|
  Terminator : Terminator
  Transfer Fcn1 : TransferFcn  Denominator=[10 1]
  Transfer Fcn2 : TransferFcn  Denominator=[10 1]
  Zero-Order Hold{1..4} (4 alike) : ZeroOrderHold  SampleTime=0.2
  Nadir measured position in Body Frame : Outport
  wires:
  Demux/3 -> Acos1/1
  Constant3/1 -> Sum/3, Sum1/1  "mounting error"
  Sum3/1 -> Sum/2  "x_body - x_lvlh angular difference along y"
  Sum4/1 -> Sum1/2  "x_body - x_lvlh angular difference along z"
  Sum/1 -> Pinhole camera model/1(In1)
  Sum1/1 -> Pinhole camera model/2(In2)
  Constant1/1 -> Sum3/2, Sum4/1
  Inverse pinhole camera model/1(Out1) -> Sin/1  "Measured x_body - x_lvlh angular difference along y"
  Inverse pinhole camera model/2(Out2) -> Sin1/1  "Measured x_body - x_lvlh angular difference along x"
  Radians to Degrees/1 -> Sum3/1
  Acos/1 -> Radians to Degrees/1  "x_body-y_lvlh angle"
  Radians to Degrees1/1 -> Sum4/2
  Acos1/1 -> Radians to Degrees1/1  "x_body-z_lvlh angle"
  Attitude B\L/1 -> Matrix Multiply/1
  Demux/2 -> Acos/1
  Constant/1 -> Matrix Multiply/2  "Earth center direction in LVLH"
  Demux/1 -> Terminator/1
  Matrix Multiply/1 -> Demux/1  "Earth center relative direction in Body Frame"
  Constant2/1 -> Sum2/1
  Square/1 -> Sum2/2
  Square1/1 -> Sum2/3
  Sum2/1 -> Sqrt/1
  Sqrt/1 -> Mux/1
  Mux/1 -> Nadir measured position in Body Frame/1, Scope/1
  Sin1/1 -> Zero-Order Hold4/1
  Sin/1 -> Zero-Order Hold1/1
  Pinhole camera model/1(Out1) -> Quantizer/1
  Pinhole camera model/2(Out2) -> Quantizer1/1
  Gain1/1 -> Sum1/3  "0.3 degree accuracy at 1 sigma"
  Band-Limited White Noise1/1 -> Gain1/1
  Band-Limited White Noise2/1 -> Gain2/1
  Gain2/1 -> Sum/1  "0.3 degree accuracy at 1 sigma"
  Transfer Fcn1/1 -> Zero-Order Hold3/1
  Quantizer/1 -> Inverse pinhole camera model/1(In1)
  Quantizer1/1 -> Inverse pinhole camera model/2(In2)
  Zero-Order Hold2/1 -> Square/1, Mux/2
  Zero-Order Hold3/1 -> Square1/1, Mux/3
  Transfer Fcn2/1 -> Zero-Order Hold2/1
  Zero-Order Hold1/1 -> Transfer Fcn2/1
  Zero-Order Hold4/1 -> Transfer Fcn1/1

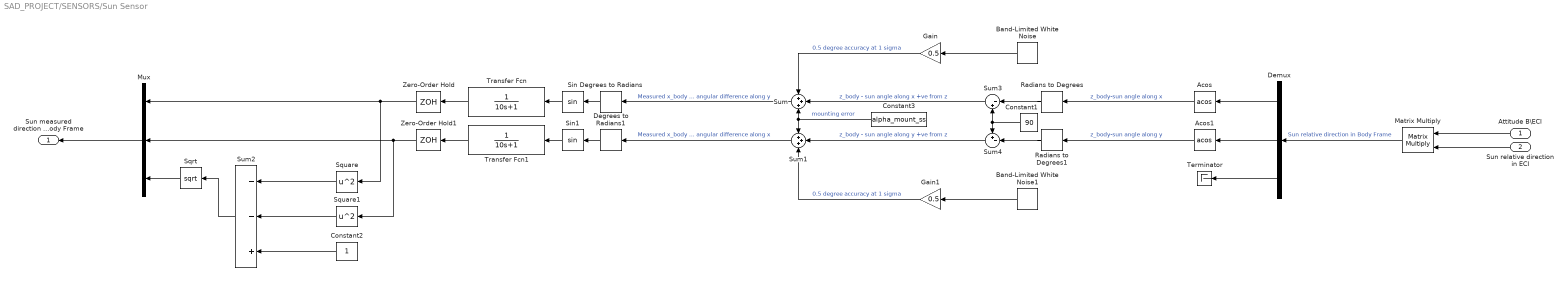
== system SAD_PROJECT/SENSORS/Sun Sensor ==
  Attitude B\ECI : Inport
  Sun relative direction in ECI : Inport  Port=2
  Acos : Trigonometry  Operator=acos
  Acos1 : Trigonometry  Operator=acos
  Band-Limited White Noise : simulink/Sources/Band-Limited White Noise  Cov=[0.1]  Ts=0.1  seed=[23341]
  Band-Limited White Noise1 : simulink/Sources/Band-Limited White Noise  Cov=[0.1]  Ts=0.1  seed=[23344]
  Constant1 : Constant  Value=90
  Constant2 : Constant
  Constant3 : Constant  Value=alpha_mount_ss
  Degrees to Radians : simulink_extras/Transformations/Degrees to Radians
  Degrees to Radians1 : simulink_extras/Transformations/Degrees to Radians
  Demux : Demux  Outputs=3
  Gain : Gain  Gain=0.5
  Gain1 : Gain  Gain=0.5
  Matrix Multiply : Product  Multiplication=Matrix(*)
  Mux : Mux  Inputs=3
  Radians to Degrees : simulink_extras/Transformations/Radians to Degrees
  Radians to Degrees1 : simulink_extras/Transformations/Radians to Degrees
  Sin : Trigonometry
  Sin1 : Trigonometry
  Sqrt : Sqrt
  Square : Math  Operator=square
  Square1 : Math  Operator=square
  Sum : Sum  Inputs=+++
  Sum1 : Sum  Inputs=+++
  Sum2 : Sum  Inputs=--+
  Sum3 : Sum  Inputs=|-+
  Sum4 : Sum  Inputs=+-|
  Terminator : Terminator
  Transfer Fcn : TransferFcn  Denominator=[10 1]
  Transfer Fcn1 : TransferFcn  Denominator=[10 1]
  Zero-Order Hold : ZeroOrderHold  SampleTime=0.2
  Zero-Order Hold1 : ZeroOrderHold  SampleTime=0.2
  Sun measured direction in Body Frame : Outport
  wires:
  Attitude B\ECI/1 -> Matrix Multiply/1
  Sin1/1 -> Transfer Fcn1/1
  Square/1 -> Sum2/1
  Square1/1 -> Sum2/2
  Sum2/1 -> Sqrt/1
  Radians to Degrees/1 -> Sum3/1
  Acos1/1 -> Radians to Degrees1/1  "z_body-sun angle along y"
  Constant1/1 -> Sum3/2, Sum4/1
  Acos/1 -> Radians to Degrees/1  "z_body-sun angle along x"
  Sum3/1 -> Sum/2  "z_body - sun angle along x +ve from z"
  Radians to Degrees1/1 -> Sum4/2
  Sum4/1 -> Sum1/2  "z_body - sun angle along y +ve from z"
  Constant3/1 -> Sum1/1, Sum/3  "mounting error"
  Sin/1 -> Transfer Fcn/1
  Matrix Multiply/1 -> Demux/1  "Sun relative direction in Body Frame"
  Demux/1 -> Acos/1
  Demux/2 -> Acos1/1
  Demux/3 -> Terminator/1
  Constant2/1 -> Sum2/3
  Sqrt/1 -> Mux/3
  Sun relative direction in ECI/1 -> Matrix Multiply/2
  Mux/1 -> Sun measured direction in Body Frame/1
  Degrees to Radians/1 -> Sin/1
  Sum/1 -> Degrees to Radians/1  "Measured x_body - x_lvlh angular difference along y"
  Degrees to Radians1/1 -> Sin1/1
  Sum1/1 -> Degrees to Radians1/1  "Measured x_body - x_lvlh angular difference along x"
  Band-Limited White Noise/1 -> Gain/1
  Gain/1 -> Sum/1  "0.5 degree accuracy at 1 sigma"
  Gain1/1 -> Sum1/3  "0.5 degree accuracy at 1 sigma"
  Band-Limited White Noise1/1 -> Gain1/1
  Transfer Fcn/1 -> Zero-Order Hold/1
  Transfer Fcn1/1 -> Zero-Order Hold1/1
  Zero-Order Hold/1 -> Square/1, Mux/1
  Zero-Order Hold1/1 -> Square1/1, Mux/2

== system SAD_PROJECT/TRIAD/Subsystem ==
  a : Inport
  b : Inport  Port=2
  Cross Product1 : matrix_library/Cross Product
  Cross Product3 : matrix_library/Cross Product
  Divide3 : Product  Inputs=*/
  Dot Product3 : DotProduct  OutDataTypeStr=Inherit: Inherit via internal rule
  Matrix Concatenate1 : Concatenate  NumInputs=3  Mode=Multidimensional array  ConcatenateDimension=2
  Sqrt4 : Sqrt
  Measures in Body : Outport
  wires:
  Matrix Concatenate1/1 -> Measures in Body/1  "Measures in Body"
  Sqrt4/1 -> Divide3/2
  Divide3/1 -> Cross Product1/2, Matrix Concatenate1/2
  Cross Product3/1 -> Dot Product3/1, Dot Product3/2, Divide3/1
  Dot Product3/1 -> Sqrt4/1
  Cross Product1/1 -> Matrix Concatenate1/3
  a/1 -> Cross Product3/1, Cross Product1/1, Matrix Concatenate1/1
  b/1 -> Cross Product3/2

== system SAD_PROJECT/TRIAD/Subsystem1 ==
  Att_LVLH/ECI : Inport
  Sun relative direction ECI : Inport  Port=2
  Matrix Multiply : Product  Multiplication=Matrix(*)
  Sun direction in LVLH : Outport
  wires:
  Att_LVLH/ECI/1 -> Matrix Multiply/1
  Sun relative direction ECI/1 -> Matrix Multiply/2
  Matrix Multiply/1 -> Sun direction in LVLH/1

== system SAD_PROJECT/TRIAD/Subsystem2 ==
  Nadir in LVLH : Inport
  Sun in LVLH : Inport  Port=2
  Cross Product2 : matrix_library/Cross Product
  Cross Product5 : matrix_library/Cross Product
  Divide1 : Product  Inputs=*/
  Dot Product1 : DotProduct  OutDataTypeStr=Inherit: Inherit via internal rule
  Matrix Concatenate : Concatenate  NumInputs=3  Mode=Multidimensional array  ConcatenateDimension=2
  Sqrt2 : Sqrt
  Transpose : Math  Operator=transpose
  Out1 : Outport
  wires:
  Nadir in LVLH/1 -> Cross Product5/1, Matrix Concatenate/1, Cross Product2/1
  Dot Product1/1 -> Sqrt2/1
  Cross Product5/1 -> Dot Product1/1, Dot Product1/2, Divide1/1
  Divide1/1 -> Cross Product2/2, Matrix Concatenate/2  "v2"
  Matrix Concatenate/1 -> Transpose/1  "Measures in LVLH"
  Cross Product2/1 -> Matrix Concatenate/3  "v3"
  Transpose/1 -> Out1/1
  Sqrt2/1 -> Divide1/2
  Sun in LVLH/1 -> Cross Product5/2

== system SAD_PROJECT/DESATURATION CONTROL LOGIC/RW 1 Desaturation/RW BRAKING ==
  In1 : Inport
  Constant8 : Constant  Value=M_brake
  Gain1 : Gain  Gain=-1
  Product : Product
  Sign : Signum
  M_braking : Outport
  wires:
  Product/1 -> M_braking/1
  Gain1/1 -> Product/2
  Constant8/1 -> Product/1
  Sign/1 -> Gain1/1
  In1/1 -> Sign/1

== system SAD_PROJECT/DESATURATION CONTROL LOGIC/RW 2 Desaturation/RW BRAKING ==
  In1 : Inport
  Constant8 : Constant  Value=M_brake
  Gain1 : Gain  Gain=-1
  Product : Product
  Sign : Signum
  M_braking : Outport
  wires:
  Product/1 -> M_braking/1
  Gain1/1 -> Product/2
  Constant8/1 -> Product/1
  Sign/1 -> Gain1/1
  In1/1 -> Sign/1

== system SAD_PROJECT/DESATURATION CONTROL LOGIC/RW 3 Desaturation/RW BRAKING ==
  In1 : Inport
  Constant8 : Constant  Value=M_brake
  Gain1 : Gain  Gain=-1
  Product : Product
  Sign : Signum
  M_braking : Outport
  wires:
  Product/1 -> M_braking/1
  Gain1/1 -> Product/2
  Constant8/1 -> Product/1
  Sign/1 -> Gain1/1
  In1/1 -> Sign/1

== system SAD_PROJECT/ENVIRONMENT/Gravity Gradient/Subsystem ==
  Att_B\L : Inport
  I_Body : Inport  Port=2
  Matrix Multiply3 : Product  Multiplication=Matrix(*)
  Matrix Multiply4 : Product  Multiplication=Matrix(*)
  Transpose2 : Math  Operator=transpose
  I LVLH FRAME : Outport
  wires:
  Matrix Multiply3/1 -> I LVLH FRAME/1  "I LVLH FRAME"
  Matrix Multiply4/1 -> Matrix Multiply3/1
  I_Body/1 -> Matrix Multiply4/2
  Att_B\L/1 -> Transpose2/1, Matrix Multiply3/2
  Transpose2/1 -> Matrix Multiply4/1

== system SAD_PROJECT/ENVIRONMENT/Magnetic Torque/Cartesian 2 spherical ==
  "[km]" : Inport
  Asin : Trigonometry  Operator=asin
  Atan2 : Trigonometry  Operator=atan2
  Constant : Constant  Value=2*pi
  Constant1 : Constant  Value=2*pi
  Constant2 : Constant  Value=2*pi
  Demux : Demux  Outputs=3
  Divide : Product  Inputs=*/
  Dot Product : DotProduct  OutDataTypeStr=Inherit: Inherit via internal rule
  Mod : Math  Operator=mod
  Mod1 : Math  Operator=mod
  Mod2 : Math  Operator=mod
  Sqrt : Sqrt
  Subsystem : Subsystem
  Subtract : Sum  Inputs=+-
  Sum : Sum  Inputs=++|
  LST : Outport
  Long : Outport  Port=2
  radius : Outport  Port=3
  lat : Outport  Port=4
  wires:
  "[km]"/1 -> Dot Product/2, Dot Product/1, Demux/1  "r_vec"
  Demux/2 -> Atan2/1  "r_y"
  Demux/1 -> Atan2/2  "r_x"
  Subsystem/1(Output) -> Sum/2, Subtract/2
  Dot Product/1 -> Sqrt/1
  Demux/3 -> Divide/1  "r_z"
  Sqrt/1 -> radius/1, Divide/2  "r"
  Divide/1 -> Asin/1
  Asin/1 -> lat/1  "latitude"
  Constant1/1 -> Mod1/2
  Subtract/1 -> Mod1/1  "longitude"
  Mod/1 -> Subtract/1
  Atan2/1 -> Mod/1  "alpha"
  Constant/1 -> Mod/2
  Mod1/1 -> Long/1, Sum/1  "longitude"
  Sum/1 -> Mod2/1
  Constant2/1 -> Mod2/2
  Mod2/1 -> LST/1

== system SAD_PROJECT/ENVIRONMENT/Magnetic Torque/MAGNETIC TORQUE in BODY ==
  local siderial time : Inport
  longitude : Inport  Port=2
  r : Inport  Port=3
  latitude : Inport  Port=4
  True_Att_B\N : Inport  Port=5
  a : Inport  Port=6
  B : Concatenate  NumInputs=3
  B in ECI system : Subsystem
  Cross Product : matrix_library/Cross Product
  Gain : Gain  Gain=1e-9
  Matrix Multiply : Product  Multiplication=Matrix(*)
  M : Outport
  Mag_fld : Outport  Port=2
  wires:
  B in ECI system/1(Out1) -> B/1
  a/1 -> Cross Product/1
  B in ECI system/2(Out2) -> B/2
  r/1 -> B in ECI system/3(r)
  local siderial time/1 -> B in ECI system/1(local siderial time)
  latitude/1 -> B in ECI system/4(latitude)
  B in ECI system/3(Out3) -> B/3
  Cross Product/1 -> M/1
  longitude/1 -> B in ECI system/2(longitude)
  B/1 -> Gain/1
  True_Att_B\N/1 -> Matrix Multiply/1
  Gain/1 -> Matrix Multiply/2
  Matrix Multiply/1 -> Mag_fld/1, Cross Product/2

== system SAD_PROJECT/NAVIGATION/S//C Orbit propagation/J2 perturbation ==
  Position vector : Inport
  Constant7 : Constant  Value=-3.5
  Demux : Demux  Outputs=3
  Dot Product1 : DotProduct  OutDataTypeStr=Inherit: Inherit via internal rule
  Gain1 : Gain  Gain=[1;1;3]
  Gain2 : Gain  Gain=1.5*J2*mu_E*R_E_eqtr^2
  Gain3 : Gain  Gain=5
  Power2 : Math  Operator=pow
  Power3 : Math  Operator=square
  Product2 : Product
  Product4 : Product
  Sum1 : Sum  Inputs=|-+
  Terminator : Terminator
  Terminator1 : Terminator
  J2 acceleration : Outport
  wires:
  Gain3/1 -> Sum1/2
  Power2/1 -> Gain2/1
  Dot Product1/1 -> Power2/1, Gain1/1  "r^2"
  Demux/1 -> Terminator/1
  Gain1/1 -> Sum1/1
  Gain2/1 -> Product2/1
  Demux/3 -> Power3/1
  Power3/1 -> Gain3/1
  Product4/1 -> Product2/2
  Demux/2 -> Terminator1/1
  Constant7/1 -> Power2/2
  Product2/1 -> J2 acceleration/1
  Position vector/1 -> Demux/1, Product4/2, Dot Product1/2, Dot Product1/1
  Sum1/1 -> Product4/1

== system SAD_PROJECT/NAVIGATION/S//C Orbit propagation/Keplerian motion ==
  Position vector : Inport
  Constant : Constant  Value=-1.5
  Dot Product2 : DotProduct  OutDataTypeStr=Inherit: Inherit via internal rule
  Gain1 : Gain  Gain=mu_E
  Power : Math  Operator=pow
  Product1 : Product
  Keplerian acceleration : Outport
  wires:
  Position vector/1 -> Product1/2, Dot Product2/2, Dot Product2/1
  Power/1 -> Gain1/1
  Gain1/1 -> Product1/1
  Product1/1 -> Keplerian acceleration/1
  Constant/1 -> Power/2
  Dot Product2/1 -> Power/1  "r^2"

== system SAD_PROJECT/NAVIGATION/Sun orbit propagation/Keplerian motion ==
  Position vector : Inport
  Constant4 : Constant  Value=-1.5
  Dot Product2 : DotProduct  OutDataTypeStr=Inherit: Inherit via internal rule
  Gain : Gain  Gain=mu_S
  Power : Math  Operator=pow
  Product1 : Product
  Keplerian acceleration : Outport
  wires:
  Position vector/1 -> Product1/2, Dot Product2/2, Dot Product2/1
  Product1/1 -> Keplerian acceleration/1
  Constant4/1 -> Power/2
  Dot Product2/1 -> Power/1  "r^2"
  Power/1 -> Gain/1
  Gain/1 -> Product1/1

== system SAD_PROJECT/OBSERVER + NOMINAL CONTROLLER/NOMINAL CONTROL/NADIR POINTING CONTROL ==
  x_hat : Inport
  Action Port : ActionPort  ActionPortLabel=else
  Gain4 : Gain  Gain=K  Multiplication=Matrix(K*u) (u vector)
  Out1 : Outport
  wires:
  Gain4/1 -> Out1/1
  x_hat/1 -> Gain4/1

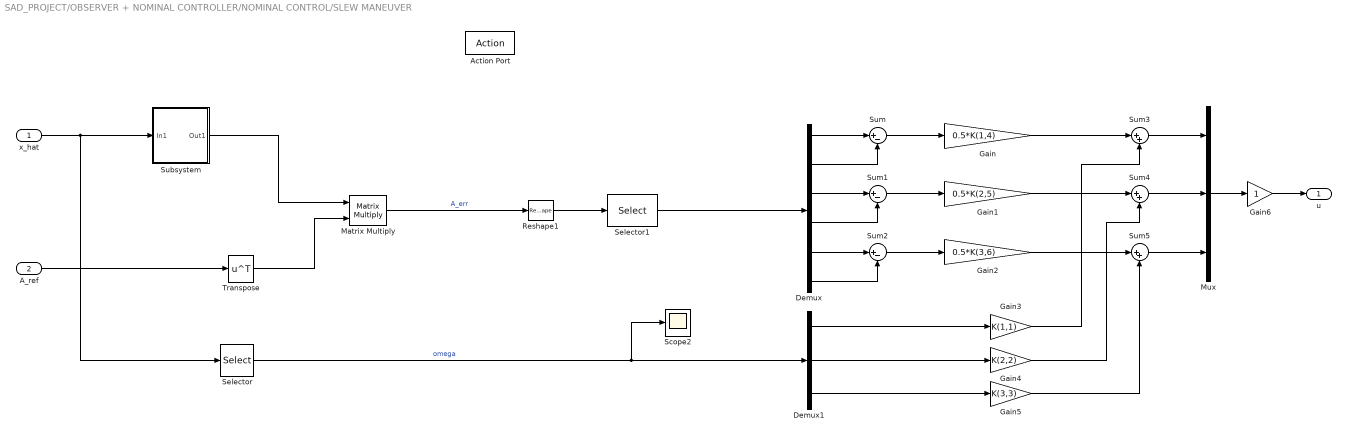
== system SAD_PROJECT/OBSERVER + NOMINAL CONTROLLER/NOMINAL CONTROL/SLEW MANEUVER ==
  x_hat : Inport
  A_ref : Inport  Port=2
  Action Port : ActionPort  ActionPortLabel=if(u1 == 3)
  Demux : Demux  Outputs=6
  Demux1 : Demux  Outputs=3
  Gain : Gain  Gain=0.5*K(1,4)
  Gain1 : Gain  Gain=0.5*K(2,5)
  Gain2 : Gain  Gain=0.5*K(3,6)
  Gain3 : Gain  Gain=K(1,1)
  Gain4 : Gain  Gain=K(2,2)
  Gain5 : Gain  Gain=K(3,3)
  Gain6 : Gain
  Matrix Multiply : Product  Multiplication=Matrix(*)
  Mux : Mux  Inputs=3
  Reshape1 : Reshape
  Scope2 : Scope
  Selector : Selector  InputPortWidth=6  IndexOptions=Index vector (dialog)  Indices=[1 2 3]  OutputSizes=1
  Selector1 : Selector  InputPortWidth=9  IndexOptions=Index vector (dialog)  Indices=[8 6 3 7 4 2]  OutputSizes=1
  Subsystem : Subsystem
  Sum : Sum  Inputs=|+-
  Sum1 : Sum  Inputs=|+-
  Sum2 : Sum  Inputs=|+-
  Sum3 : Sum  Inputs=|++
  Sum4 : Sum  Inputs=|++
  Sum5 : Sum  Inputs=|++
  Transpose : Math  Operator=transpose
  u : Outport
  wires:
  x_hat/1 -> Selector/1, Subsystem/1(In1)
  A_ref/1 -> Transpose/1
  Transpose/1 -> Matrix Multiply/2
  Matrix Multiply/1 -> Reshape1/1  "A_err"
  Reshape1/1 -> Selector1/1
  Selector1/1 -> Demux/1
  Demux/2 -> Sum/2
  Demux/4 -> Sum1/2
  Demux/1 -> Sum/1
  Demux/3 -> Sum1/1
  Demux/6 -> Sum2/2
  Demux/5 -> Sum2/1
  Sum/1 -> Gain/1
  Sum1/1 -> Gain1/1
  Sum2/1 -> Gain2/1
  Demux1/1 -> Gain3/1
  Demux1/2 -> Gain4/1
  Demux1/3 -> Gain5/1
  Gain/1 -> Sum3/1
  Gain1/1 -> Sum4/1
  Gain2/1 -> Sum5/1
  Gain3/1 -> Sum3/2
  Gain4/1 -> Sum4/2
  Gain5/1 -> Sum5/2
  Sum3/1 -> Mux/1
  Sum4/1 -> Mux/2
  Sum5/1 -> Mux/3
  Mux/1 -> Gain6/1
  Selector/1 -> Scope2/1, Demux1/1  "omega"
  Gain6/1 -> u/1
  Subsystem/1(Out1) -> Matrix Multiply/1
